simulink model "HevMmPowertrainController"  (R2022b)
settings: configuration reference "VehicleFixed10ms" (kept outside this file)
undefined symbols (not defined in the file): CtrlVcuHevMmBattChrgPwrMax, CtrlVcuHevMmBattDischrgPwrMax, CtrlVcuHevMmChrgLmtBpt, CtrlVcuHevMmCSChrgFctr, CtrlVcuHevMmDischrgLmtBpt, CtrlVcuHevMmEngPwr, CtrlVcuHevMmEngSpd, CtrlVcuHevMmEngTrq, CtrlVcuHevMmN_idle, CtrlVcuHevMmRegenBrkCutOff, CtrlVcuHevMmRegenBrkSpdBpt, CtrlVcuHevMmSocBpt, CtrlVcuHevMmSOCChrgFctr, CtrlVcuHevMmSOCmax, CtrlVcuHevMmSOCmin, CtrlVcuHevMmSOCtarget, DiscIntNeverNeededParam, PlntBattChrgMax, PlntBrkActrBoreFrnt, PlntBrkFrntBias, PlntBrkKinFricCffFrnt, PlntBrkNumPadsFrnt, PlntBrkPadMeanRadiusFrnt, PlntBrkPrsFctr, PlntBrkRearBias, PlntDiffrntlRatio, PlntEM1EffTbl, PlntEM1Spd, PlntEM1Trq, PlntEM1TrqEff, PlntEM2EffTbl, PlntEM2Spd, PlntEM2Trq, PlntEM2TrqEff, PlntHevMmGenGearRatio, PlntHevMmMotGearRatio, PlntVehMass, PlntWhlLdRadius
libraries: simulink x15, autolibutils x1
(part 2 of 2)

== stateflow chart HevMmPowertrainController/Multi-Mode_Hybrid_Control ==
  state ChargeSustain_Mode
    during:
    PwrCmd = MotTrqCmd*MotSpd;
    SOCopt = (SOCTrgt/100) - 0.5*VehMass*VehSpd*VehSpd*CSChrgFctr/BattEnrgy;
    ChrgPwr = SOCChrgFctr*(SOCopt - SOC/100);
    state CSModes [parallel]
      du:
      [EVArea,EngArea,EVPwr_bound,EVSpdmax] = OperatingAreaCalc(VehSpd,SOC,PwrCmd);
      settings: executionOrder=1
      state HEV
        en:
        HEVMode=1;
        CSMode = 2;
        ex:
        HEVMode=0;
        state Temporal_Logic
          state start
          (default) -> ChargeSustain_Mode.CSModes.HEV.Temporal_Logic.start
          (junction 270) -> ChargeSustain_Mode.CSModes.HEV.Temporal_Logic.start [order 2] : [EVArea==0 && EngArea==0]
          (junction 272) -> ChargeSustain_Mode.CSModes.HEV.Temporal_Logic.start [order 2] : [EVArea==0 && EngArea==0]
          ChargeSustain_Mode.CSModes.HEV.Temporal_Logic.start -> (junction 272) [order 2] : [EVArea==1 && EngArea==0]
          ChargeSustain_Mode.CSModes.HEV.Temporal_Logic.start -> (junction 270) [order 1] : [EVArea==0 && EngArea==1]
        (default) -> ChargeSustain_Mode.CSModes.HEV.Temporal_Logic
      state Note [group]
        note: In Charge Sustain Mode, you can operate in
            | EV, HEV, or Engine Modes.
            |
            | The embedded SL function is using Force requested
            | and Vehicle Speed to determine if you are operating
            | in the EV Area or Engine Area.  If you are not in either
            | area then you are in the HEV Area.
            |
            | If SOC drops below 30% you will be forced into HEV mode
            | if in the other 2 modes.  There is temporal logic in place
            | to make sure you don't jump between modes too quickly.
      note: after(5, sec)...
          |  &&[SOC > SOCTrgt]
      note: after(5, sec)...
          |  && [SOC > SOCTrgt]
      state EV
        en:
        EVMode=1;
        CSMode = 1;
        ex:
        EVMode=0;
        state Temporal_Logic
          state start
          (junction 255) -> ChargeSustain_Mode.CSModes.EV.Temporal_Logic.start [order 2] : [EVArea==1 && EngArea==0]
          (default) -> ChargeSustain_Mode.CSModes.EV.Temporal_Logic.start
          ChargeSustain_Mode.CSModes.EV.Temporal_Logic.start -> (junction 255) [order 1] : [EVArea==0 && EngArea==0]
          ChargeSustain_Mode.CSModes.EV.Temporal_Logic.start -> (junction 254) [order 2] : [EVArea==0 && EngArea==1]
          (junction 254) -> ChargeSustain_Mode.CSModes.EV.Temporal_Logic.start [order 2] : [EVArea==1 && EngArea==0]
        (default) -> ChargeSustain_Mode.CSModes.EV.Temporal_Logic
      state Eng
        en:
        EngMode=1;
        CSMode = 3;
        ex:
        EngMode=0;
        state Temporal_Logic
          state start
          (junction 304) -> ChargeSustain_Mode.CSModes.Eng.Temporal_Logic.start [order 2] : [EVArea==0 && EngArea==1]
          ChargeSustain_Mode.CSModes.Eng.Temporal_Logic.start -> (junction 304) [order 2] : [EVArea==0 && EngArea==0]
          (default) -> ChargeSustain_Mode.CSModes.Eng.Temporal_Logic.start
          ChargeSustain_Mode.CSModes.Eng.Temporal_Logic.start -> (junction 302) [order 1] : [EVArea==1 && EngArea==0]
          (junction 302) -> ChargeSustain_Mode.CSModes.Eng.Temporal_Logic.start [order 2] : [EVArea==0 && EngArea==1]
        (default) -> ChargeSustain_Mode.CSModes.Eng.Temporal_Logic
      state [EVArea,EngArea,EVPwr_bound,EVSpdmax] = OperatingAreaCalc(VehSpd,SOC,PwrCmd) [function]
      (junction 254) -> ChargeSustain_Mode.CSModes.Eng [order 1] : after(1.5,sec)
      (default) -> EV
      (junction 270) -> ChargeSustain_Mode.CSModes.Eng [order 1] : after(5, sec)
      (junction 272) -> EV [order 1] : after(5, sec)
      (junction 302) -> EV [order 1] : after(1.5,sec)
      (junction 255) -> ChargeSustain_Mode.CSModes.HEV [order 1] : after(1.5,sec)
      (junction 304) -> ChargeSustain_Mode.CSModes.HEV [order 1] : after(1.5,sec)
    state MotControl [parallel]
      settings: executionOrder=2
      state EV_HEV
        en, du:
        MotMode = 1;
        MotTrqCmd_init = MotTrqCmd;
      state Eng
        en, du:
        MotMode = 3;
        MotTrqCmd_init = MotTrqAssist_Req;
      (default) -> EV_HEV
      EV_HEV -> ChargeSustain_Mode.MotControl.Eng : [EngMode == 6]
      ChargeSustain_Mode.MotControl.Eng -> EV_HEV : [EngMode ~= 6]
    state Generator_Control [parallel]
      settings: executionOrder=3
      state Off
        entry, during:
        GenMode = 1;
        GenTrqCmd = 0;
      state On
        entry, during:
        GenMode = 2;
        GenTrqCmd = GenControl(EngSpd,EngSpdCmd);
        state GenTrqCmd = GenControl(EngSpd,EngSpdCmd) [function]
      (default) -> ChargeSustain_Mode.Generator_Control.Off
      On -> ChargeSustain_Mode.Generator_Control.Off : [EngMode == 6 || EngMode == 1 || ...
          |  EngMode == 5]
      ChargeSustain_Mode.Generator_Control.Off -> On : [EngMode ==2 || EngMode == 3 || ...
          | EngMode == 4]
    state Engine_Control [parallel]
      settings: executionOrder=4
      state Off
        entry, during:
        EngMode = 1;
        EngTrqCmd = 0;
        EngSpdCmd = 0;
        EngStarted = 0;
      state Starting
        entry, during:
        EngMode = 2;
        EngTrqCmd = 0;
        EngSpdCmd = EngIdle;
      state Eng
        exit:
        EngCltchCmd = 0;
        state Clutch_Close
          entry, during:
          EngMode = 4;
          EngStarted = 1;
          EngSpdCmd = EngCltchOutSpd;
          EngTrqCmd = 0;
          EngCltchCmd = ClutchControl(EngCltchOutSpd,EngSpd);
          state EngCltchCmd = ClutchControl(EngCltchOutSpd,EngSpd) [function]
        state Wait
          en, du:
          EngMode = 5;
        state Direct_Engine_Drive
          entry, during:
          EngMode = 6;
          EngStarted = 1;
          EngSpdCmd = 0;
          [EngTrqCmd,MotTrqAssist_Req] = EngTrqControl(F_req,EngSpd);
          state [EngTrqCmd,MotTrqAssist_Req] = EngTrqControl(F_req,EngSpd) [function]
        (default) -> Clutch_Close
        Clutch_Close -> Wait : [EngCltchCmd]
        Wait -> Direct_Engine_Drive : [ClutchState]
      state HEV
        entry, during:
        EngMode = 3;
        EngStarted = 1;
        [EngTrqCmd,EngSpdCmd] = TrqCalc(MotTrqCmd,MotSpd,ChrgPwr,BattPwrDischrgLmt,BattPwrChrgLmt,GenSpd,GenTrqCmd);
        state [EngTrqCmd,EngSpdCmd] = TrqCalc(MotTrqCmd,MotSpd,ChrgPwr,BattPwrDischrgLmt,BattPwrChrgLmt,GenSpd,GenTrqCmd) [function]
      (default) -> ChargeSustain_Mode.Engine_Control.Off
      ChargeSustain_Mode.Engine_Control.Off -> Starting : [CSMode == 2 ...
          |  || CSMode == 3]
      Starting -> ChargeSustain_Mode.Engine_Control.Off [order 2] : [CSMode == 1]
      ChargeSustain_Mode.Engine_Control.HEV -> ChargeSustain_Mode.Engine_Control.Off [order 1] : [CSMode == 1]
      ChargeSustain_Mode.Engine_Control.Eng -> ChargeSustain_Mode.Engine_Control.Off [order 1] : [CSMode == 1]
      Starting -> (junction 564) [order 1] : [EngSpd > 50]
      (junction 564) -> (junction 631) [order 2] : [CSMode == 3]
      (junction 631) -> ChargeSustain_Mode.Engine_Control.Eng
      (junction 564) -> ChargeSustain_Mode.Engine_Control.HEV [order 1] : [CSMode == 2]
      ChargeSustain_Mode.Engine_Control.HEV -> ChargeSustain_Mode.Engine_Control.Eng [order 2] : [CSMode == 3]
      ChargeSustain_Mode.Engine_Control.Eng -> ChargeSustain_Mode.Engine_Control.HEV [order 2] : [CSMode == 2]
  data: EVArea function_output; EngArea function_output; VehSpd function_input size=1; SOC function_input size=1; EVPwr_bound function_output; PwrCmd function_input; EVSpdmax function_output; EngSpd function_input; GenTrqCmd function_output; EngSpdCmd function_input; EngCltchOutSpd function_input; EngSpd function_input; EngCltchCmd function_output; F_req function_input; EngTrqCmd function_output; MotTrqAssist_Req function_output; EngSpd function_input; EngTrqCmd function_output; EngSpdCmd function_output; MotTrqCmd function_input; MotSpd function_input; ChrgPwr function_input; BattPwrDischrgLmt function_input; BattPwrChrgLmt function_input; GenSpd function_input; GenTrqCmd function_input; MotMode output double; EngIdle input; SOCTrgt input; VehMass input; HEVMode local double; EngStarted local boolean =0; CSChrgFctr input; BattEnrgy input; SOC input; SOCChrgFctr input; VehSpd input; ClutchState input boolean; EngSpd input; EVArea local boolean; EngArea local boolean; EVMode local double; EngCltchOutSpd input; MotSpd input; GenSpd input; BattPwrChrgLmt input; BattPwrDischrgLmt input; F_req input; CSMode output double; MotTrqAssist_Req output single; EngMode output double; GenMode output double; EngSpdCmd output double; ChrgPwr output double; PwrCmd output double; EVPwr_bound output double; EVSpdmax output double; EngCltchCmd output [0..1] =0; EngTrqCmd output; GenTrqCmd output =0; MotTrqCmd input; MotTrqCmd_init output double; SOCopt local double
